simulink model "gm_combinedTxRx_AXIMM"  (R2017b)
settings: Solver=FixedStepDiscrete  StartTime=0.0  StopTime=10.0  RelTol=1e-3
InitFcn:
  | modelSettings
undefined symbols (not defined in the file or in its folder): coeff, filt, j, RadioSampleRate, VibertiTracebackLength, xPreambleSeq
libraries: hdlmdlgenlib x24, simulink x20, dsphdlfiltering x20, hdlsllib x10, dspsigops x5, commseqgen3 x4, commdigbbndpm3 x3, commcrc2 x2, commcnvcod2 x2, commsource2 x1, dspstat3 x1, dspmlti4 x1
(part 3 of 6)

== system gm_combinedTxRx_AXIMM/Combined TX and RX/Receiver HDL/Frame Recover/Barker Locate/Measure Phase Ambiguity ==
  data : Inport  OutDataTypeStr=int16  SampleTime=1e-06
  trigger : Inport  Port=2  SampleTime=1e-06
  validIn : Inport  Port=3  SampleTime=1e-06
  Find Max and Set Output Shift : Subsystem
  HDL Opt Complex FIR4 : Subsystem  mask{Taps=reshape([complex(-0.7071067811865477, -0.7071067811865475) complex(-0.7071067811865477, -0.7071067811865475) complex(-0.7071067811865477, -0.7071067811865475) complex(0.7071067811865476, 0.7071067811865476) complex(0.7071067811865476, 0.7071067811865476) complex(0.7071067811865476, 0.7071067811865476) complex(-0.7071067811865477, -0.7071067811865475) complex(0.7071067811865476, 0.7071067811865476) complex(-0.7071067811865477, -0.7071067811865475) complex(-0.7071067811865477, -0.7071067811865475) complex(0.7071067811865476, 0.7071067811865476) complex(-0.7071067811865477, -0.7071067811865475) complex(-0.7071067811865477, -0.7071067811865475) complex(-0.7071067811865477, -0.7071067811865475) complex(0.7071067811865476, 0.7071067811865476) complex(0.7071067811865476, 0.7071067811865476) complex(0.7071067811865476, 0.7071067811865476) complex(-0.7071067811865477, -0.7071067811865475) complex(0.7071067811865476, 0.7071067811865476) complex(-0.7071067811865477, -0.7071067811865475) complex(-0.7071067811865477, -0.7071067811865475) complex(0.7071067811865476, 0.7071067811865476) complex(-0.7071067811865477, -0.7071067811865475) complex(-0.7071067811865477, -0.7071067811865475) complex(-0.7071067811865477, -0.7071067811865475) complex(0.7071067811865476, 0.7071067811865476) complex(0.7071067811865476, 0.7071067811865476) complex(0.7071067811865476, 0.7071067811865476)].', [1  28])}
  HDL Opt Complex FIR5 : Subsystem  mask{Taps=reshape([complex(-0.7071067811865475, 0.7071067811865477) complex(-0.7071067811865475, 0.7071067811865477) complex(-0.7071067811865475, 0.7071067811865477) complex(0.7071067811865476, -0.7071067811865476) complex(0.7071067811865476, -0.7071067811865476) complex(0.7071067811865476, -0.7071067811865476) complex(-0.7071067811865475, 0.7071067811865477) complex(0.7071067811865476, -0.7071067811865476) complex(-0.7071067811865475, 0.7071067811865477) complex(-0.7071067811865475, 0.7071067811865477) complex(0.7071067811865476, -0.7071067811865476) complex(-0.7071067811865475, 0.7071067811865477) complex(-0.7071067811865475, 0.7071067811865477) complex(-0.7071067811865475, 0.7071067811865477) complex(0.7071067811865476, -0.7071067811865476) complex(0.7071067811865476, -0.7071067811865476) complex(0.7071067811865476, -0.7071067811865476) complex(-0.7071067811865475, 0.7071067811865477) complex(0.7071067811865476, -0.7071067811865476) complex(-0.7071067811865475, 0.7071067811865477) complex(-0.7071067811865475, 0.7071067811865477) complex(0.7071067811865476, -0.7071067811865476) complex(-0.7071067811865475, 0.7071067811865477) complex(-0.7071067811865475, 0.7071067811865477) complex(-0.7071067811865475, 0.7071067811865477) complex(0.7071067811865476, -0.7071067811865476) complex(0.7071067811865476, -0.7071067811865476) complex(0.7071067811865476, -0.7071067811865476)].', [1  28])}
  HDL Opt Complex FIR6 : Subsystem  mask{Taps=reshape([complex(0.7071067811865476, 0.7071067811865476) complex(0.7071067811865476, 0.7071067811865476) complex(0.7071067811865476, 0.7071067811865476) complex(-0.7071067811865475, -0.7071067811865477) complex(-0.7071067811865475, -0.7071067811865477) complex(-0.7071067811865475, -0.7071067811865477) complex(0.7071067811865476, 0.7071067811865476) complex(-0.7071067811865475, -0.7071067811865477) complex(0.7071067811865476, 0.7071067811865476) complex(0.7071067811865476, 0.7071067811865476) complex(-0.7071067811865475, -0.7071067811865477) complex(0.7071067811865476, 0.7071067811865476) complex(0.7071067811865476, 0.7071067811865476) complex(0.7071067811865476, 0.7071067811865476) complex(-0.7071067811865475, -0.7071067811865477) complex(-0.7071067811865475, -0.7071067811865477) complex(-0.7071067811865475, -0.7071067811865477) complex(0.7071067811865476, 0.7071067811865476) complex(-0.7071067811865475, -0.7071067811865477) complex(0.7071067811865476, 0.7071067811865476) complex(0.7071067811865476, 0.7071067811865476) complex(-0.7071067811865475, -0.7071067811865477) complex(0.7071067811865476, 0.7071067811865476) complex(0.7071067811865476, 0.7071067811865476) complex(0.7071067811865476, 0.7071067811865476) complex(-0.7071067811865475, -0.7071067811865477) complex(-0.7071067811865475, -0.7071067811865477) complex(-0.7071067811865475, -0.7071067811865477)].', [1  28])}
  HDL Opt Complex FIR7 : Subsystem  mask{Taps=reshape([complex(0.7071067811865476, -0.7071067811865476) complex(0.7071067811865476, -0.7071067811865476) complex(0.7071067811865476, -0.7071067811865476) complex(-0.7071067811865477, 0.7071067811865475) complex(-0.7071067811865477, 0.7071067811865475) complex(-0.7071067811865477, 0.7071067811865475) complex(0.7071067811865476, -0.7071067811865476) complex(-0.7071067811865477, 0.7071067811865475) complex(0.7071067811865476, -0.7071067811865476) complex(0.7071067811865476, -0.7071067811865476) complex(-0.7071067811865477, 0.7071067811865475) complex(0.7071067811865476, -0.7071067811865476) complex(0.7071067811865476, -0.7071067811865476) complex(0.7071067811865476, -0.7071067811865476) complex(-0.7071067811865477, 0.7071067811865475) complex(-0.7071067811865477, 0.7071067811865475) complex(-0.7071067811865477, 0.7071067811865475) complex(0.7071067811865476, -0.7071067811865476) complex(-0.7071067811865477, 0.7071067811865475) complex(0.7071067811865476, -0.7071067811865476) complex(0.7071067811865476, -0.7071067811865476) complex(-0.7071067811865477, 0.7071067811865475) complex(0.7071067811865476, -0.7071067811865476) complex(0.7071067811865476, -0.7071067811865476) complex(0.7071067811865476, -0.7071067811865476) complex(-0.7071067811865477, 0.7071067811865475) complex(-0.7071067811865477, 0.7071067811865475) complex(-0.7071067811865477, 0.7071067811865475)].', [1  28])}
  Logical Operator : Logic  Inputs=5  AllPortsSameDT=off  OutDataTypeStr=boolean  SampleTime=1e-06
  delayMatch{,1..3} (4 alike) : Delay  DelayLength=hex2num('4010000000000000')  InitialCondition=0  InputProcessing=Inherited  SampleTime=1e-06
  PA : Outport  InitialOutput=0
  wires:
  Find Max and Set Output Shift/1(Out1) -> PA/1
  HDL Opt Complex FIR4/1(Out1) -> Find Max and Set Output Shift/1(In1)
  delayMatch/1 -> Logical Operator/1
  HDL Opt Complex FIR5/1(Out1) -> Find Max and Set Output Shift/2(In2)
  delayMatch1/1 -> Logical Operator/2
  HDL Opt Complex FIR6/1(Out1) -> Find Max and Set Output Shift/3(In4)
  delayMatch2/1 -> Logical Operator/3
  HDL Opt Complex FIR7/1(Out1) -> Find Max and Set Output Shift/4(In5)
  delayMatch3/1 -> Logical Operator/4
  Logical Operator/1 -> Find Max and Set Output Shift/5(Enable)
  data/1 -> HDL Opt Complex FIR4/1(In1), HDL Opt Complex FIR5/1(In1), HDL Opt Complex FIR7/1(In1), HDL Opt Complex FIR6/1(In1)
  trigger/1 -> Logical Operator/5
  validIn/1 -> HDL Opt Complex FIR4/2(validIn), HDL Opt Complex FIR5/2(validIn), HDL Opt Complex FIR7/2(validIn), HDL Opt Complex FIR6/2(validIn)
  HDL Opt Complex FIR4/2(validOut) -> delayMatch/1
  HDL Opt Complex FIR5/2(validOut) -> delayMatch1/1
  HDL Opt Complex FIR6/2(validOut) -> delayMatch2/1
  HDL Opt Complex FIR7/2(validOut) -> delayMatch3/1

== system gm_combinedTxRx_AXIMM/Combined TX and RX/Receiver HDL/Frame Recover/Equalization and Demodulation/2 Bit Descrambler ==
  note: This is a special Descrambler which can process 2 bits at a time
  u1 : Inport  PortDimensions=2  SampleTime=1e-06
  reset : Inport  Port=2  SampleTime=1e-06
  Enable_out4 : Inport  Port=3  OutDataTypeStr=boolean  SampleTime=1e-06
  MATLAB Function : Subsystem
      settings: MinAlgLoopOccurrences=on
  Selector1 : Selector  SampleTime=1e-06  IndexOptions=Index vector (dialog)  Indices=[hex2num('3ff0000000000000') hex2num('4008000000000000') hex2num('4014000000000000') hex2num('401c000000000000')]  OutputSizes=hex2num('3ff0000000000000')
  Selector2 : Selector  SampleTime=1e-06  IndexOptions=Index vector (dialog)  Indices=[hex2num('3ff0000000000000') hex2num('4008000000000000') hex2num('4014000000000000') hex2num('401c000000000000')]  OutputSizes=hex2num('3ff0000000000000')
  delayMatch : Delay  DelayLength=hex2num('4000000000000000')  InitialCondition=0  InputProcessing=Inherited
  input_xor1 : Logic  Operator=XOR  AllPortsSameDT=off  OutDataTypeStr=boolean  SampleTime=1e-06
  input_xor2 : Logic  Operator=XOR  AllPortsSameDT=off  OutDataTypeStr=boolean  SampleTime=1e-06
  mux : Mux  Inputs=2
  state_xor1 : Logic  Operator=XOR  Inputs=1  AllPortsSameDT=off  OutDataTypeStr=boolean  SampleTime=1e-06
  state_xor2 : Logic  Operator=XOR  Inputs=1  AllPortsSameDT=off  OutDataTypeStr=boolean  SampleTime=1e-06
  t : Demux  Outputs=2
  u1_0_wire : hdlmdlgenlib/Buffer
      settings: SourceProductName=HDL Coder  SourceProductBaseCode=HD
  u1_1_wire : hdlmdlgenlib/Buffer
      settings: SourceProductName=HDL Coder  SourceProductBaseCode=HD
  y1 : Outport  InitialOutput=0
  wires:
  u1_0_wire/1 -> input_xor1/2
  u1_1_wire/1 -> input_xor2/2
  MATLAB Function/1(out0) -> Selector1/1
  MATLAB Function/2(out1) -> Selector2/1
  mux/1 -> y1/1
  Selector1/1 -> state_xor1/1
  Selector2/1 -> state_xor2/1
  input_xor1/1 -> mux/1
  input_xor2/1 -> mux/2
  state_xor1/1 -> input_xor1/1
  state_xor2/1 -> input_xor2/1
  delayMatch/1 -> MATLAB Function/Enable
  t/1 -> u1_0_wire/1
  t/2 -> u1_1_wire/1
  u1/1 -> t/1, MATLAB Function/1(in0)
  reset/1 -> MATLAB Function/2(in1)
  Enable_out4/1 -> delayMatch/1

== system gm_combinedTxRx_AXIMM/Combined TX and RX/Receiver HDL/Frame Recover/Equalization and Demodulation/Align with Start ==
  in0 : Inport  OutDataTypeStr=boolean  SampleTime=1e-06
  Enable_out4 : EnablePort  OutDataTypeStr=boolean
  Align with Start : Delay  DelayLength=hex2num('3ff0000000000000')  InitialCondition=0  InputProcessing=Inherited
  out0 : Outport  OutDataTypeStr=boolean  InitialOutput=0
  wires:
  Align with Start/1 -> out0/1
  in0/1 -> Align with Start/1

== system gm_combinedTxRx_AXIMM/Combined TX and RX/Receiver HDL/Frame Recover/Equalization and Demodulation/DFE ==
  note: Generate training sequence when barker is found
  note: refTap=0 to disableEQ
  Trigger : Inport  PortDimensions=1  SampleTime=1e-06
  data : Inport  Port=2  PortDimensions=1  SampleTime=1e-06
      settings: SignalType=complex
  EQmu : Inport  Port=3  SampleTime=1e-06
  Enable_out4 : Inport  Port=4  OutDataTypeStr=boolean  SampleTime=1e-06
  DFE : Subsystem  mask{numFTaps=hex2num('4014000000000000'), numBTaps=hex2num('4008000000000000'), mu=hex2num('3f847ae147ae147b'), refTap=hex2num('4000000000000000')}
      mask prompts: numFTaps "Num Forward Taps"; numBTaps "Num Backward Taps"; mu "Step Size"; refTap "Reference Tap"
  Delay data so DFE can reset : Subsystem
      settings: MinAlgLoopOccurrences=on
  Delay ref so DFE can reset : Subsystem
      settings: MinAlgLoopOccurrences=on
  PN Sequence Generator : Subsystem
      settings: MinAlgLoopOccurrences=on
  Packeted To Unpacked : Subsystem
  QPSK Modulator Baseband : Subsystem
      settings: MinAlgLoopOccurrences=on
  Terminator1 : Terminator
  delayMatch : Delay  DelayLength=hex2num('4000000000000000')  InitialCondition=0  InputProcessing=Inherited
  dataEQed : Outport  InitialOutput=0
  start : Outport  Port=2  InitialOutput=0
  wires:
  DFE/1(eqOut) -> dataEQed/1
  DFE/2(err) -> Terminator1/1
  DFE/3(start) -> start/1
  Delay data so DFE can reset/1(out0) -> DFE/2(dataIn)
  Delay ref so DFE can reset/1(out0) -> DFE/3(training)
  PN Sequence Generator/1(out0) -> Packeted To Unpacked/1(In1)
  Packeted To Unpacked/1(Out1) -> QPSK Modulator Baseband/1(in0)
  QPSK Modulator Baseband/1(out0) -> Delay ref so DFE can reset/1(in0)
  delayMatch/1 -> Delay data so DFE can reset/Enable
  Trigger/1 -> PN Sequence Generator/1(in0), DFE/1(reset)
  data/1 -> Delay data so DFE can reset/1(in0)
  EQmu/1 -> DFE/4(EQmu)
  Enable_out4/1 -> delayMatch/1, QPSK Modulator Baseband/Enable, PN Sequence Generator/Enable, Delay ref so DFE can reset/Enable, DFE/5(Enable_out4)

== system gm_combinedTxRx_AXIMM/Combined TX and RX/Receiver HDL/Frame Recover/Equalization and Demodulation/Header Controller ==
  in0 : Inport  OutDataTypeStr=boolean  SampleTime=1e-06
  in1 : Inport  Port=2  OutDataTypeStr=boolean  PortDimensions=[2]  SampleTime=1e-06
  Enable_out4 : EnablePort  OutDataTypeStr=boolean
  Header Controller : Subsystem
  out0 : Outport  OutDataTypeStr=boolean  InitialOutput=0
  out1 : Outport  Port=2  OutDataTypeStr=uint16  InitialOutput=0
  out2 : Outport  Port=3  OutDataTypeStr=boolean  InitialOutput=0
  out3 : Outport  Port=4  OutDataTypeStr=boolean  InitialOutput=0
  out4 : Outport  Port=5  OutDataTypeStr=uint8  InitialOutput=0
  out5 : Outport  Port=6  OutDataTypeStr=uint32  InitialOutput=0
  out6 : Outport  Port=7  OutDataTypeStr=uint32  InitialOutput=0
  wires:
  Header Controller/1(enableDownstream) -> out0/1
  Header Controller/2(packetLenBitsOut) -> out1/1
  Header Controller/3(resetViterbi) -> out2/1
  Header Controller/4(crcStart) -> out3/1
  Header Controller/5(status) -> out4/1
  Header Controller/6(s1) -> out5/1
  Header Controller/7(s2) -> out6/1
  in0/1 -> Header Controller/1(headerStart)
  in1/1 -> Header Controller/2(data)

== system gm_combinedTxRx_AXIMM/Combined TX and RX/Receiver HDL/Frame Recover/Equalization and Demodulation/QPSK Demodulator Baseband ==
  in0 : Inport  OutDataTypeStr=fixdt(1, 16, 14)  SampleTime=1e-06
      settings: SignalType=complex
  Enable_out4 : EnablePort  OutDataTypeStr=boolean
  QPSK Demodulator Baseband : commdigbbndpm3/QPSK Demodulator Baseband  OutType=Bit  DecType=Hard decision  VarSource=Dialog  Variance=1  Dec=Binary  Ph=pi/4  outDtype1=boolean  outDtype2=Inherit via internal rule  derotateFactorWordLen=16  derotateFactorDataTypeStr=Inherit: Same word length as input  derotateFactorLastDataTypeStr=Inherit: Same word length as input
  out0 : Outport  OutDataTypeStr=boolean  PortDimensions=[2]  InitialOutput=0
  wires:
  QPSK Demodulator Baseband/1 -> out0/1
  in0/1 -> QPSK Demodulator Baseband/1

== system gm_combinedTxRx_AXIMM/Combined TX and RX/Receiver HDL/Frame Recover/Equalization and Demodulation/Skip EQ Training Symbols After Barker ==
  in0 : Inport  OutDataTypeStr=boolean  SampleTime=1e-06
  Enable_out4 : EnablePort  OutDataTypeStr=boolean
  Skip EQ Training Symbols After Barker : Delay  DelayLength=hex2num('406f400000000000')  InitialCondition=0  InputProcessing=Inherited
  out0 : Outport  OutDataTypeStr=boolean  InitialOutput=0
  wires:
  Skip EQ Training Symbols After Barker/1 -> out0/1
  in0/1 -> Skip EQ Training Symbols After Barker/1

== system gm_combinedTxRx_AXIMM/Combined TX and RX/Receiver HDL/Frame Recover/Frequency Recovery/Delay ==
  in0 : Inport  OutDataTypeStr=fixdt(1, 16, 13)  SampleTime=1e-06
      settings: SignalType=complex
  Enable_out4 : EnablePort  OutDataTypeStr=boolean
  Delay : Delay  DelayLength=hex2num('3ff0000000000000')  InitialCondition=0  InputProcessing=Inherited
  out0 : Outport  OutDataTypeStr=fixdt(1, 16, 13)  InitialOutput=0
      settings: SignalType=complex
  wires:
  Delay/1 -> out0/1
  in0/1 -> Delay/1

== system gm_combinedTxRx_AXIMM/Combined TX and RX/Receiver HDL/Frame Recover/Frequency Recovery/Lock Detector ==
  ped : Inport  SampleTime=1e-06
  Enable_out4 : Inport  Port=2  OutDataTypeStr=boolean  SampleTime=1e-06
  Compare To Constant : simulink/Logic and Bit Operations/Compare To Constant  relop=<=  const=fi(0,0,23,10,'hex','000c00')  OutDataTypeStr=boolean
  MATLAB Function : Subsystem
  Pipeline Delay : Subsystem
      settings: MinAlgLoopOccurrences=on
  Sum of Elements : Sum  Inputs=+  AccumDataTypeStr=fixdt(0, 23, 10)  OutDataTypeStr=fixdt(0, 23, 10)  SampleTime=1e-06
  Tapped Delay : Subsystem
      settings: MinAlgLoopOccurrences=on
  lock : Outport  InitialOutput=0
  wires:
  Compare To Constant/1 -> lock/1
  MATLAB Function/1(y) -> Tapped Delay/1(in0)
  Pipeline Delay/1(out0) -> MATLAB Function/1(u)
  Sum of Elements/1 -> Compare To Constant/1
  Tapped Delay/1(out0) -> Sum of Elements/1
  ped/1 -> Pipeline Delay/1(in0)
  Enable_out4/1 -> Tapped Delay/Enable, Pipeline Delay/Enable

== system gm_combinedTxRx_AXIMM/Combined TX and RX/Receiver HDL/Frame Recover/Frequency Recovery/Loop Filter Configurable ==
  note: This inflation is necessary
  e : Inport  SampleTime=1e-06
  LoopBW : Inport  Port=2  SampleTime=1e-06
  Enable_out4 : Inport  Port=3  OutDataTypeStr=boolean  SampleTime=1e-06
  Add1 : Sum  AccumDataTypeStr=fixdt(1, 17, 10)  OutDataTypeStr=fixdt(1, 16, 10)  RndMeth=Nearest  SampleTime=1e-06
  Add2 : Sum  AccumDataTypeStr=fixdt(1, 17, 10)  OutDataTypeStr=fixdt(1, 16, 10)  SampleTime=1e-06
  Data Type Conversion : DataTypeConversion  OutDataTypeStr=fixdt(1, 25, 20)  SampleTime=1e-06
  Delay : Subsystem
      settings: MinAlgLoopOccurrences=on
  Delay3 : Subsystem
      settings: MinAlgLoopOccurrences=on
  Delay4 : Subsystem
      settings: MinAlgLoopOccurrences=on
  Direct Lookup Table (n-D) : LookupNDDirect  NumberOfTableDimensions=1  Table="reshape([0.038055419921875;0.074676513671875;0.109954833984375;0.143951416015625;0.1767578125;0.208404541015625;0.23895263671875;0.268463134765625;0.296966552734375;0.324554443359375;0.351226806640625;0.3770751953125;0.402069091796875;0.426300048828125;0.44976806640625;0.472564697265625;0.49462890625;0.51605224609375;0.536865234375;0.55706787109375;0.576690673828125;0.59576416015625;0.614288330078125;0.63232421875;0.64984130859375;0.666900634765625;0.683502197265625;0.699676513671875;0.715423583984375;0.730743408203125;0.745697021484375;0.76025390625;0.774444580078125;0.788299560546875;0.801788330078125;0.814971923828125;0.82781982421875;0.840362548828125;0.85260009765625;0.86456298828125;0.876251220703125;0.887664794921875;0.8988037109375;0.909698486328125;0.92034912109375;0.930755615234375;0.94091796875;0.950897216796875;0.96063232421875;0.97015380859375;0.979461669921875;0.98858642578125;0.99749755859375;1.006256103515625;1.014801025390625;1.023162841796875;1.0313720703125;1.0394287109375;1.047271728515625;1.05499267578125;1.06256103515625;1.0699462890625;1.07720947265625;1.084320068359375;1.09130859375;1.09814453125;1.1048583984375;1.111419677734375;1.117889404296875;1.12420654296875;1.130401611328125;1.136505126953125;1.142486572265625;1.148345947265625;1.154083251953125;1.159759521484375;1.165283203125;1.170745849609375;1.17608642578125;1.18133544921875;1.18646240234375;1.1915283203125;1.196502685546875;1.201385498046875;1.2061767578125;1.21087646484375;1.21551513671875;1.220062255859375;1.224517822265625;1.228912353515625;1.23321533203125;1.237457275390625;1.241607666015625;1.2457275390625;1.249725341796875;1.253692626953125;1.257568359375;1.26141357421875;1.265167236328125;1.26885986328125;1.272491455078125;1.27606201171875;1.279571533203125;1.28302001953125;1.286407470703125;1.289764404296875;1.29302978515625;1.2962646484375;1.2994384765625;1.302581787109375;1.3056640625;1.308685302734375;1.3116455078125;1.3145751953125;1.317474365234375;1.3203125;1.323089599609375;1.325836181640625;1.328521728515625;1.3311767578125;1.33380126953125;1.33636474609375;1.338897705078125;1.341400146484375;1.343841552734375;1.34625244140625;1.3486328125;1.350982666015625], [128    1])"  DiagnosticForOutOfRangeInput=Error  SampleTime=1e-06  TableDataTypeStr=fixdt('ufix16_En15')
  Direct Lookup Table (n-D)1 : LookupNDDirect  NumberOfTableDimensions=1  Table="reshape([1.1444091796875e-05;4.482269287109375e-05;0.00010013580322265625;0.00017452239990234375;0.00026798248291015625;0.00037860870361328125;0.00050640106201171875;0.0006504058837890625;0.00080966949462890625;0.00098323822021484375;0.001171112060546875;0.0013713836669921875;0.00158405303955078125;0.00180816650390625;0.002044677734375;0.0022907257080078125;0.0025482177734375;0.00281524658203125;0.00309085845947265625;0.003376007080078125;0.00366973876953125;0.00397205352783203125;0.00428104400634765625;0.0045986175537109375;0.0049228668212890625;0.0052547454833984375;0.00559234619140625;0.00593662261962890625;0.00628662109375;0.0066432952880859375;0.00700473785400390625;0.0073719024658203125;0.00774478912353515625;0.008121490478515625;0.00850391387939453125;0.0088901519775390625;0.009281158447265625;0.00967693328857421875;0.0100765228271484375;0.01047992706298828125;0.01088619232177734375;0.0112972259521484375;0.01171207427978515625;0.0121288299560546875;0.01255035400390625;0.012973785400390625;0.013401031494140625;0.01383113861083984375;0.01426410675048828125;0.01469898223876953125;0.01513671875;0.0155773162841796875;0.01602077484130859375;0.0164661407470703125;0.01691341400146484375;0.0173625946044921875;0.01781463623046875;0.018268585205078125;0.0187244415283203125;0.0191822052001953125;0.01964092254638671875;0.02010250091552734375;0.020565032958984375;0.02102947235107421875;0.021495819091796875;0.0219631195068359375;0.0224323272705078125;0.02290248870849609375;0.02337360382080078125;0.02384662628173828125;0.0243206024169921875;0.02479648590087890625;0.02527332305908203125;0.0257511138916015625;0.0262298583984375;0.02670955657958984375;0.02719020843505859375;0.02767181396484375;0.0281543731689453125;0.02863788604736328125;0.02912235260009765625;0.0296077728271484375;0.030094146728515625;0.0305805206298828125;0.03106784820556640625;0.03155612945556640625;0.0320453643798828125;0.03253459930419921875;0.03302478790283203125;0.03351593017578125;0.03400707244873046875;0.03449916839599609375;0.03499126434326171875;0.03548431396484375;0.03597736358642578125;0.03647136688232421875;0.03696537017822265625;0.03745937347412109375;0.0379543304443359375;0.0384502410888671875;0.03894519805908203125;0.0394420623779296875;0.0399379730224609375;0.04043483734130859375;0.04093170166015625;0.04142856597900390625;0.0419254302978515625;0.042423248291015625;0.0429210662841796875;0.04341888427734375;0.04391765594482421875;0.04441547393798828125;0.04491424560546875;0.04541301727294921875;0.0459117889404296875;0.04641056060791015625;0.046909332275390625;0.04740810394287109375;0.04790782928466796875;0.0484066009521484375;0.0489063262939453125;0.04940509796142578125;0.04990482330322265625;0.05040454864501953125;0.0509033203125;0.051403045654296875;0.05190181732177734375;0.05240154266357421875], [128    1])"  DiagnosticForOutOfRangeInput=Error  SampleTime=1e-06  TableDataTypeStr=fixdt('ufix16_En20')
  Product : Product  Inputs=**  OutDataTypeStr=fixdt(1, 16, 10)  SampleTime=1e-06
  Product1 : Product  Inputs=**  OutDataTypeStr=fixdt(1, 16, 10)  SampleTime=1e-06
  Sum2 : Sum  AccumDataTypeStr=fixdt(1, 17, 10)  OutDataTypeStr=fixdt(1, 16, 10)  SampleTime=1e-06
  v : Outport  InitialOutput=0
  wires:
  e/1 -> Product1/1, Product/1
  LoopBW/1 -> Direct Lookup Table (n-D)1/1, Direct Lookup Table (n-D)/1
  Add1/1 -> Sum2/2
  Add2/1 -> Data Type Conversion/1, Delay4/1(in0)
  Data Type Conversion/1 -> v/1
  Delay/1(out0) -> Add1/1
  Delay3/1(out0) -> Add2/1
  Delay4/1(out0) -> Add2/2
  Direct Lookup Table (n-D)/1 -> Product/2
  Direct Lookup Table (n-D)1/1 -> Product1/2
  Product/1 -> Sum2/1
  Product1/1 -> Add1/2, Delay/1(in0)
  Sum2/1 -> Delay3/1(in0)
  Enable_out4/1 -> Delay4/Enable, Delay3/Enable, Delay/Enable

== system gm_combinedTxRx_AXIMM/Combined TX and RX/Receiver HDL/Frame Recover/Frequency Recovery/PED ==
  In : Inport  SampleTime=1e-06
  RxTxFixedPointLibrary_c16_PED : MATLAB Function  TreatAsAtomicUnit=on
  e : Outport  InitialOutput=0
  wires:
  In/1 -> RxTxFixedPointLibrary_c16_PED/1(In)
  RxTxFixedPointLibrary_c16_PED/1(e) -> e/1

== system gm_combinedTxRx_AXIMM/Combined TX and RX/Receiver HDL/Frame Recover/Frequency Recovery/Phase Shift FP ==
  In1 : Inport  SampleTime=1e-06
  Phi : Inport  Port=2  SampleTime=1e-06
  Cosine HDL Optimized : hdlsllib/Lookup Tables/Cosine HDL Optimized  OutputFormula=exp(j*2*pi*u)  NumDataPoints=256  TableDataTypeStr=fixdt(0,31,20)  SimulateLUTROMDelay=off
      settings: SourceProductName=HDL Coder  SourceProductBaseCode=HD
  Gain : Gain  Gain=fi(0,1,25,20,'hex','1fd741a')  ParamDataTypeStr=fixdt(1, 25, 20)  OutDataTypeStr=fixdt(1, 16, 12)  SampleTime=1e-06  SaturateOnIntegerOverflow=on
  Product{,1..3} (4 alike) : Product  Inputs=**  OutDataTypeStr=fixdt(1, 16, 13)  SampleTime=1e-06  SaturateOnIntegerOverflow=on
  Product_AC_minus_BD : Sum  Inputs=+-  OutDataTypeStr=fixdt(1, 16, 13)  SampleTime=1e-06  SaturateOnIntegerOverflow=on
  Product_AD_plus_BC : Sum  OutDataTypeStr=fixdt(1, 16, 13)  SampleTime=1e-06  SaturateOnIntegerOverflow=on
  Product_C2ReIm_1 : ComplexToRealImag  SampleTime=1e-06
  Product_C2ReIm_2 : ComplexToRealImag  SampleTime=1e-06
  Product_ReIm2Complex : RealImagToComplex  SampleTime=1e-06
  Out1 : Outport  InitialOutput=0
  wires:
  In1/1 -> Product_C2ReIm_1/1
  Phi/1 -> Gain/1
  Cosine HDL Optimized/1 -> Product_C2ReIm_2/1
  Gain/1 -> Cosine HDL Optimized/1
  Product_ReIm2Complex/1 -> Out1/1
  Product_C2ReIm_1/1 -> Product1/1, Product/1
  Product_C2ReIm_1/2 -> Product3/1, Product2/1
  Product_C2ReIm_2/1 -> Product3/2, Product/2
  Product_C2ReIm_2/2 -> Product2/2, Product1/2
  Product/1 -> Product_AC_minus_BD/1
  Product1/1 -> Product_AD_plus_BC/1
  Product2/1 -> Product_AC_minus_BD/2
  Product3/1 -> Product_AD_plus_BC/2
  Product_AC_minus_BD/1 -> Product_ReIm2Complex/1
  Product_AD_plus_BC/1 -> Product_ReIm2Complex/2

== system gm_combinedTxRx_AXIMM/Combined TX and RX/Receiver HDL/Frame Recover/Gardner Timing Recovery/Delay ==
  in0 : Inport  OutDataTypeStr=fixdt(0, 15, 14)  SampleTime=1e-06
  Enable_out2 : EnablePort  OutDataTypeStr=boolean
  Delay : Delay  DelayLength=hex2num('3ff0000000000000')  InitialCondition=0  InputProcessing=Inherited
  out0 : Outport  OutDataTypeStr=fixdt(0, 15, 14)  InitialOutput=0
  wires:
  Delay/1 -> out0/1
  in0/1 -> Delay/1

== system gm_combinedTxRx_AXIMM/Combined TX and RX/Receiver HDL/Frame Recover/Gardner Timing Recovery/Delay1 ==
  in0 : Inport  OutDataTypeStr=boolean  SampleTime=1e-06
  Enable_out2 : EnablePort  OutDataTypeStr=boolean
  Delay1 : Delay  DelayLength=hex2num('3ff0000000000000')  InitialCondition=0  InputProcessing=Inherited
  out0 : Outport  OutDataTypeStr=boolean  InitialOutput=0
  wires:
  Delay1/1 -> out0/1
  in0/1 -> Delay1/1

== system gm_combinedTxRx_AXIMM/Combined TX and RX/Receiver HDL/Frame Recover/Gardner Timing Recovery/Delay2 ==
  in0 : Inport  OutDataTypeStr=fixdt(1, 16, 13)  SampleTime=1e-06
      settings: SignalType=complex
  Enable_out2 : EnablePort  OutDataTypeStr=boolean
  Delay2 : Delay  DelayLength=hex2num('4018000000000000')  InitialCondition=0  InputProcessing=Inherited
  out0 : Outport  OutDataTypeStr=fixdt(1, 16, 13)  InitialOutput=0
      settings: SignalType=complex
  wires:
  Delay2/1 -> out0/1
  in0/1 -> Delay2/1

== system gm_combinedTxRx_AXIMM/Combined TX and RX/Receiver HDL/Frame Recover/Gardner Timing Recovery/Gardner TED Blocks ==
  note: This is for QPSK and 4 SamplesPerSymbol ONLY
  data : Inport  SampleTime=1e-06
  strobe : Inport  Port=2  SampleTime=1e-06
  Enable_out2 : Inport  Port=3  OutDataTypeStr=boolean  SampleTime=1e-06
  Add : Sum  AccumDataTypeStr=fixdt(1, 33, 20)  OutDataTypeStr=fixdt(1, 16, 15)  SampleTime=1e-06
  Check Only Strobe Condition : simulink/Logic and Bit Operations/Compare To Constant  relop===  const=fi(0,1,8,0,'hex','01')  OutDataTypeStr=boolean
  Complex to Real-Imag : ComplexToRealImag  SampleTime=1e-06
  Constant : Constant  Value=fi(0,1,16,15,'hex','0000')  OutDataTypeStr=fixdt(1, 16, 15)  SampleTime=-1
  Display : Display
  Imag Error : Subsystem
  Logical Operator : Logic  AllPortsSameDT=off  OutDataTypeStr=boolean  SampleTime=1e-06
  Map [0,1,2,3,4] to [0,1,2,2,2] : LookupNDDirect  NumberOfTableDimensions=1  Table="reshape([hex2num('0000000000000000') hex2num('3ff0000000000000') hex2num('4000000000000000') hex2num('4000000000000000') hex2num('4000000000000000')].', [1  5])"  DiagnosticForOutOfRangeInput=Error  SampleTime=1e-06  TableDataTypeStr=uint8
  Real Error : Subsystem
  Strobe Buffer1_tap1 : Subsystem
      settings: MinAlgLoopOccurrences=on
  Strobe Buffer1_tap2 : Subsystem
      settings: MinAlgLoopOccurrences=on
  Strobe Buffer1_tap3 : Subsystem
      settings: MinAlgLoopOccurrences=on
  Sum of Elements1 : Sum  Inputs=+  AccumDataTypeStr=fixdt(0, 10, 0)  OutDataTypeStr=int8  SampleTime=1e-06
  Switch : Switch  Criteria=u2 ~= 0  Threshold=hex2num('0000000000000000')  OutDataTypeStr=fixdt(1, 16, 15)  SampleTime=1e-06  SaturateOnIntegerOverflow=on
  t : Mux
  e : Outport  InitialOutput=0
  wires:
  data/1 -> Complex to Real-Imag/1
  strobe/1 -> Logical Operator/2, Strobe Buffer1_tap1/1(in0), t/4
  Add/1 -> Switch/1
  Check Only Strobe Condition/1 -> Logical Operator/1
  Complex to Real-Imag/1 -> Real Error/1(data)
  Complex to Real-Imag/2 -> Imag Error/1(data)
  Constant/1 -> Switch/3
  Imag Error/1(Out1) -> Add/2
  Logical Operator/1 -> Switch/2
  Map [0,1,2,3,4] to [0,1,2,2,2]/1 -> Imag Error/2(strobe sum), Real Error/2(strobe sum)
  Real Error/1(Out1) -> Add/1
  t/1 -> Sum of Elements1/1
  Sum of Elements1/1 -> Map [0,1,2,3,4] to [0,1,2,2,2]/1, Check Only Strobe Condition/1, Display/1
  Switch/1 -> e/1
  Strobe Buffer1_tap1/1(out0) -> Strobe Buffer1_tap2/1(in0), t/3
  Strobe Buffer1_tap2/1(out0) -> Strobe Buffer1_tap3/1(in0), t/2
  Strobe Buffer1_tap3/1(out0) -> t/1
  Enable_out2/1 -> Strobe Buffer1_tap3/Enable, Strobe Buffer1_tap2/Enable, Strobe Buffer1_tap1/Enable, Real Error/3(Enable_out2), Imag Error/3(Enable_out2)

== system gm_combinedTxRx_AXIMM/Combined TX and RX/Receiver HDL/Frame Recover/Gardner Timing Recovery/InterpControl_Blocks1 ==
  note: Mu is always positive
  note: e<<1/SPS
  e : Inport  SampleTime=1e-06
  Enable_out2 : Inport  Port=2  OutDataTypeStr=boolean  SampleTime=1e-06
  1/SPS1 : Constant  Value=fi(0,0,2,2,'hex','1')  OutDataTypeStr=fixdt(0, 2, 2)  SampleTime=-1
  Add1 : Sum  AccumDataTypeStr=fixdt(1, 25, 24)  OutDataTypeStr=fixdt(0, 16, 16)  SampleTime=1e-06
  Calculate New mu : Subsystem
  Display{,1..3} (4 alike) : Display
  Mod 1 : Subsystem
  NCOCounter State : Subsystem
      settings: MinAlgLoopOccurrences=on
  Subtract1 : Sum  Inputs=-+  AccumDataTypeStr=fixdt(1, 17, 16)  OutDataTypeStr=fixdt(0, 16, 16)  SampleTime=1e-06
  Update mu on strobe : Switch  Criteria=u2 > Threshold  Threshold=hex2num('0000000000000000')  OutDataTypeStr=fixdt(0, 15, 14)  SampleTime=1e-06
  saved mu : Subsystem
      settings: MinAlgLoopOccurrences=on
  strobe == W>NCOCounter : RelationalOperator  Operator=>  OutDataTypeStr=boolean  SampleTime=1e-06  RndMeth=Nearest
  strobe : Outport  InitialOutput=0
  mu : Outport  Port=2  InitialOutput=0
  wires:
  e/1 -> Add1/1
  1/SPS1/1 -> Add1/2
  Add1/1 -> strobe == W>NCOCounter/1, Subtract1/1, Display2/1, Calculate New mu/1(W)
  Calculate New mu/1(mu) -> Update mu on strobe/1, Display/1
  Mod 1/1(Out1) -> NCOCounter State/1(in0)
  NCOCounter State/1(out0) -> strobe == W>NCOCounter/2, Subtract1/2, Display1/1, Calculate New mu/2(NCOCounter)
  Subtract1/1 -> Mod 1/1(In1)
  Update mu on strobe/1 -> saved mu/1(in0), Display3/1, mu/1
  saved mu/1(out0) -> Update mu on strobe/3
  strobe == W>NCOCounter/1 -> Update mu on strobe/2, strobe/1
  Enable_out2/1 -> saved mu/Enable, NCOCounter State/Enable

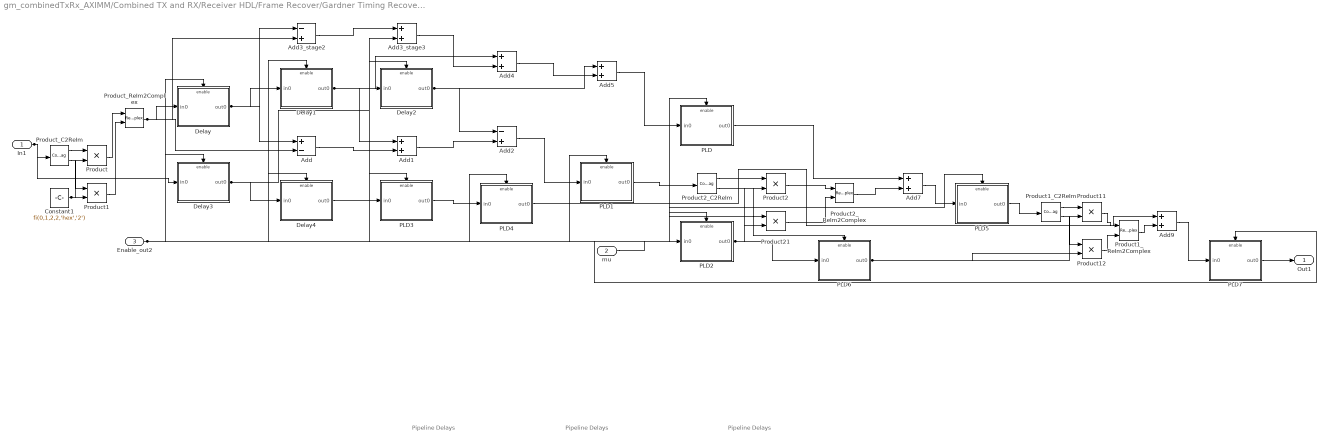
== system gm_combinedTxRx_AXIMM/Combined TX and RX/Receiver HDL/Frame Recover/Gardner Timing Recovery/Interpolator ==
  note: Pipeline Delays
  note: Pipeline Delays
  note: Pipeline Delays
  In1 : Inport  SampleTime=1e-06
  mu : Inport  Port=2  SampleTime=1e-06
  Enable_out2 : Inport  Port=3  OutDataTypeStr=boolean  SampleTime=1e-06
  Add : Sum  Inputs=+-  AccumDataTypeStr=fixdt(1, 17, 14)  OutDataTypeStr=fixdt(1, 16, 14)  SampleTime=1e-06
  Add1 : Sum  AccumDataTypeStr=fixdt(1, 17, 14)  OutDataTypeStr=fixdt(1, 17, 14)  SampleTime=1e-06
  Add2 : Sum  Inputs=-+  AccumDataTypeStr=fixdt(1, 18, 14)  OutDataTypeStr=fixdt(1, 18, 14)  SampleTime=1e-06
  Add3_stage2 : Sum  Inputs=-+  AccumDataTypeStr=fixdt(1, 18, 14)  OutDataTypeStr=fixdt(1, 18, 14)  SampleTime=1e-06
  Add3_stage3 : Sum  AccumDataTypeStr=fixdt(1, 18, 14)  OutDataTypeStr=fixdt(1, 18, 14)  SampleTime=1e-06
  Add4 : Sum  AccumDataTypeStr=fixdt(1, 19, 14)  OutDataTypeStr=fixdt(1, 19, 14)  SampleTime=1e-06
  Add5 : Sum  AccumDataTypeStr=fixdt(1, 20, 14)  OutDataTypeStr=fixdt(1, 20, 14)  SampleTime=1e-06
  Add7 : Sum  AccumDataTypeStr=fixdt(1, 21, 14)  OutDataTypeStr=fixdt(1, 21, 14)  SampleTime=1e-06
  Add9 : Sum  AccumDataTypeStr=fixdt(1, 37, 28)  OutDataTypeStr=fixdt(1, 16, 10)  SampleTime=1e-06
  Constant1 : Constant  Value=fi(0,1,2,2,'hex','2')  OutDataTypeStr=fixdt(1, 2, 2)  SampleTime=-1
  Delay : Subsystem
      settings: MinAlgLoopOccurrences=on
  Delay1 : Subsystem
      settings: MinAlgLoopOccurrences=on
  Delay2 : Subsystem
      settings: MinAlgLoopOccurrences=on
  Delay3 : Subsystem
      settings: MinAlgLoopOccurrences=on
  Delay4 : Subsystem
      settings: MinAlgLoopOccurrences=on
  PLD : Subsystem
      settings: MinAlgLoopOccurrences=on
  PLD1 : Subsystem
      settings: MinAlgLoopOccurrences=on
  PLD2 : Subsystem
      settings: MinAlgLoopOccurrences=on
  PLD3 : Subsystem
      settings: MinAlgLoopOccurrences=on
  PLD4 : Subsystem
      settings: MinAlgLoopOccurrences=on
  PLD5 : Subsystem
      settings: MinAlgLoopOccurrences=on
  PLD6 : Subsystem
      settings: MinAlgLoopOccurrences=on
  PLD7 : Subsystem
      settings: MinAlgLoopOccurrences=on
  Product : Product  Inputs=**  OutDataTypeStr=fixdt(1, 16, 14)  SampleTime=1e-06
  Product1 : Product  Inputs=**  OutDataTypeStr=fixdt(1, 16, 14)  SampleTime=1e-06
  Product11 : Product  Inputs=**  OutDataTypeStr=fixdt(1, 36, 28)  SampleTime=1e-06
  Product12 : Product  Inputs=**  OutDataTypeStr=fixdt(1, 36, 28)  SampleTime=1e-06
  Product1_C2ReIm : ComplexToRealImag  SampleTime=1e-06
  Product1_ReIm2Complex : RealImagToComplex  SampleTime=1e-06
  Product2 : Product  Inputs=**  OutDataTypeStr=fixdt(1, 16, 10)  SampleTime=1e-06
  Product21 : Product  Inputs=**  OutDataTypeStr=fixdt(1, 16, 10)  SampleTime=1e-06
  Product2_C2ReIm : ComplexToRealImag  SampleTime=1e-06
  Product2_ReIm2Complex : RealImagToComplex  SampleTime=1e-06
  Product_C2ReIm : ComplexToRealImag  SampleTime=1e-06
  Product_ReIm2Complex : RealImagToComplex  SampleTime=1e-06
  Out1 : Outport  InitialOutput=0
  wires:
  In1/1 -> Product_C2ReIm/1, Delay3/1(in0)
  mu/1 -> PLD2/1(in0)
  Add/1 -> Add1/2
  Add1/1 -> Add2/2
  Add2/1 -> PLD1/1(in0)
  Add3_stage3/1 -> Add4/2
  Add4/1 -> Add5/2
  Add5/1 -> PLD/1(in0)
  Add7/1 -> PLD5/1(in0)
  Add9/1 -> PLD7/1(in0)
  Constant1/1 -> Product1/2, Product/2
  Delay/1(out0) -> Add3_stage2/1, Add/1, Delay1/1(in0)
  Delay1/1(out0) -> Add4/1, Add1/1, Delay2/1(in0)
  Delay2/1(out0) -> Add5/1, Add2/1
  Delay3/1(out0) -> Add3_stage3/2, Delay4/1(in0)
  Delay4/1(out0) -> PLD3/1(in0)
  PLD/1(out0) -> Add7/1
  PLD1/1(out0) -> Product2_C2ReIm/1
  PLD2/1(out0) -> Product21/2, Product2/2, PLD6/1(in0)
  PLD3/1(out0) -> PLD4/1(in0)
  PLD4/1(out0) -> Add9/1
  PLD5/1(out0) -> Product1_C2ReIm/1
  PLD6/1(out0) -> Product12/2, Product11/2
  PLD7/1(out0) -> Out1/1
  Product_ReIm2Complex/1 -> Add3_stage2/2, Add/2, Delay/1(in0)
  Product1_ReIm2Complex/1 -> Add9/2
  Product2_ReIm2Complex/1 -> Add7/2
  Enable_out2/1 -> PLD7/Enable, PLD6/Enable, PLD5/Enable, PLD4/Enable, PLD3/Enable, PLD2/Enable, PLD1/Enable, PLD/Enable, Delay4/Enable, Delay3/Enable, Delay2/Enable, Delay1/Enable, Delay/Enable
  Add3_stage2/1 -> Add3_stage3/1
  Product_C2ReIm/1 -> Product/1
  Product_C2ReIm/2 -> Product1/1
  Product/1 -> Product_ReIm2Complex/1
  Product1/1 -> Product_ReIm2Complex/2
  Product1_C2ReIm/1 -> Product11/1
  Product1_C2ReIm/2 -> Product12/1
  Product11/1 -> Product1_ReIm2Complex/1
  Product12/1 -> Product1_ReIm2Complex/2
  Product2_C2ReIm/1 -> Product2/1
  Product2_C2ReIm/2 -> Product21/1
  Product2/1 -> Product2_ReIm2Complex/1
  Product21/1 -> Product2_ReIm2Complex/2

== system gm_combinedTxRx_AXIMM/Combined TX and RX/Receiver HDL/Frame Recover/Gardner Timing Recovery/LoopFilter1 ==
  e : Inport  SampleTime=1e-06
  Enable_out2 : Inport  Port=2  OutDataTypeStr=boolean  SampleTime=1e-06
  Delay1 : Subsystem
      settings: MinAlgLoopOccurrences=on
  Delay2 : Subsystem
      settings: MinAlgLoopOccurrences=on
  Proportional Gain : Gain  Gain=fi(0,1,16,23,'hex','9500')  ParamDataTypeStr=fixdt(1, 16, 23)  OutDataTypeStr=fixdt(1, 16, 24)  SampleTime=1e-06
  v : Outport  InitialOutput=0
  wires:
  e/1 -> Delay2/1(in0)
  Delay1/1(out0) -> v/1
  Delay2/1(out0) -> Proportional Gain/1
  Proportional Gain/1 -> Delay1/1(in0)
  Enable_out2/1 -> Delay2/Enable, Delay1/Enable

== system gm_combinedTxRx_AXIMM/Combined TX and RX/Receiver HDL/Frame Recover/Gardner Timing Recovery/TED Lock Detector ==
  ted : Inport  SampleTime=1e-06
  Enable_out2 : Inport  Port=2  OutDataTypeStr=boolean  SampleTime=1e-06
  Compare To Constant : simulink/Logic and Bit Operations/Compare To Constant  relop=<=  const=fi(0,0,23,15,'hex','008000')  OutDataTypeStr=boolean
  MATLAB Function : Subsystem
  Pipeline Delay : Subsystem
      settings: MinAlgLoopOccurrences=on
  Sum of Elements : Sum  Inputs=+  AccumDataTypeStr=fixdt(0, 23, 15)  OutDataTypeStr=fixdt(0, 23, 15)  SampleTime=1e-06
  Tapped Delay : Subsystem
      settings: MinAlgLoopOccurrences=on
  lock : Outport  InitialOutput=0
  wires:
  Compare To Constant/1 -> lock/1
  MATLAB Function/1(y) -> Tapped Delay/1(in0)
  Pipeline Delay/1(out0) -> MATLAB Function/1(u)
  Sum of Elements/1 -> Compare To Constant/1
  Tapped Delay/1(out0) -> Sum of Elements/1
  ted/1 -> Pipeline Delay/1(in0)
  Enable_out2/1 -> Tapped Delay/Enable, Pipeline Delay/Enable

== system gm_combinedTxRx_AXIMM/Combined TX and RX/Receiver HDL/Viterbi Decode/Buffer/MATLAB Function ==
  valid : Inport  SampleTime=1e-06
  start : Inport  Port=2  SampleTime=1e-06
  crcEnd : Inport  Port=3  SampleTime=1e-06
  RxTxFixedPointLibrary_c26_MATLAB_Function : MATLAB Function  TreatAsAtomicUnit=on
  enable : Outport
  wires:
  RxTxFixedPointLibrary_c26_MATLAB_Function/1(enable) -> enable/1
  valid/1 -> RxTxFixedPointLibrary_c26_MATLAB_Function/1(valid)
  start/1 -> RxTxFixedPointLibrary_c26_MATLAB_Function/2(start)
  crcEnd/1 -> RxTxFixedPointLibrary_c26_MATLAB_Function/3(crcEnd)

== system gm_combinedTxRx_AXIMM/Combined TX and RX/Receiver HDL/Viterbi Decode/Buffer/MATLAB Function1 ==
  packetLen : Inport  SampleTime=1e-06
  valid : Inport  Port=2  SampleTime=1e-06
  crcStart : Inport  Port=3  SampleTime=1e-06
  RxTxFixedPointLibrary_c2_MATLAB_Function1 : MATLAB Function  TreatAsAtomicUnit=on
  enablePop : Outport
  validOut : Outport  Port=2
  viterbiReset : Outport  Port=3
  crcOut : Outport  Port=4
  wires:
  RxTxFixedPointLibrary_c2_MATLAB_Function1/1(enablePop) -> enablePop/1
  RxTxFixedPointLibrary_c2_MATLAB_Function1/2(validOut) -> validOut/1
  RxTxFixedPointLibrary_c2_MATLAB_Function1/3(viterbiReset) -> viterbiReset/1
  RxTxFixedPointLibrary_c2_MATLAB_Function1/4(crcOut) -> crcOut/1
  packetLen/1 -> RxTxFixedPointLibrary_c2_MATLAB_Function1/1(packetLen)
  valid/1 -> RxTxFixedPointLibrary_c2_MATLAB_Function1/2(valid)
  crcStart/1 -> RxTxFixedPointLibrary_c2_MATLAB_Function1/3(crcStart)

== system gm_combinedTxRx_AXIMM/Combined TX and RX/Transmitter HDL/Packet Generation/Payload/HDL Scrambler 2 bits ==
  bitsIn : Inport  PortDimensions=[2, 1]  SampleTime=4e-06
  reset : Inport  Port=2  SampleTime=4e-06
  Buffer Manage : Subsystem
  Delay : Delay  DelayLength=1  InitialCondition=false
  Delay1 : Delay  DelayLength=1  InitialCondition=false
  Demux : Demux  Outputs=2
  Display1 : Display
  Display3 : Display
  Mux : Mux  Inputs=2
  Mux1 : Mux  Inputs=2
  Selector : Selector  IndexOptions=Index vector (dialog)  Indices=find(poly(2:end))  OutputSizes=1
  Selector1 : Selector  IndexOptions=Index vector (dialog)  Indices=1+find(poly(2:end))  OutputSizes=1
  state_xor1 : Logic  Operator=XOR  IconShape=distinctive  AllPortsSameDT=off  OutDataTypeStr=boolean
  state_xor2 : Logic  Operator=XOR  Inputs=1  IconShape=distinctive  AllPortsSameDT=off  OutDataTypeStr=boolean
  state_xor3 : Logic  Operator=XOR  Inputs=1  IconShape=distinctive  AllPortsSameDT=off  OutDataTypeStr=boolean
  state_xor4 : Logic  Operator=XOR  IconShape=distinctive  AllPortsSameDT=off  OutDataTypeStr=boolean
  bitsOut : Outport
  wires:
  bitsIn/1 -> Demux/1, Display1/1
  reset/1 -> Buffer Manage/3(reset)
  Buffer Manage/1(outBuffer) -> Selector/1, Mux1/1
  Delay/1 -> Buffer Manage/1(bit1)
  Delay1/1 -> Buffer Manage/2(bit2)
  Demux/1 -> state_xor1/2
  Demux/2 -> state_xor4/2
  Mux/1 -> bitsOut/1
  Mux1/1 -> Selector1/1
  Selector/1 -> state_xor2/1
  Selector1/1 -> state_xor3/1
  state_xor1/1 -> Mux1/2, Mux/1, Delay/1
  state_xor2/1 -> state_xor1/1, Display3/1
  state_xor3/1 -> state_xor4/1
  state_xor4/1 -> Mux/2, Delay1/1

== system gm_combinedTxRx_AXIMM/Combined TX and RX/Transmitter HDL/Packet Generation/Payload/MATLAB Function ==
  enable : Inport  SampleTime=4e-06
  RxTxFixedPointLibrary_c4_MATLAB_Function : MATLAB Function  TreatAsAtomicUnit=on
  reset : Outport
  mode : Outport  Port=2
  wires:
  enable/1 -> RxTxFixedPointLibrary_c4_MATLAB_Function/1(enable)
  RxTxFixedPointLibrary_c4_MATLAB_Function/1(reset) -> reset/1
  RxTxFixedPointLibrary_c4_MATLAB_Function/2(mode) -> mode/1

== system gm_combinedTxRx_AXIMM/Combined TX and RX/Transmitter HDL/Packet Generation/Payload/Subsystem ==
  In1 : Inport  SampleTime=4e-06
  In2 : Inport  Port=2  SampleTime=4e-06
  Logical Operator : Logic  Operator=OR  Inputs=3  AllPortsSameDT=off  OutDataTypeStr=boolean
  MATLAB Function3 : Subsystem
  Out1 : Outport
  wires:
  In1/1 -> Logical Operator/1, MATLAB Function3/1(start)
  In2/1 -> Logical Operator/3, MATLAB Function3/2(done)
  Logical Operator/1 -> Out1/1
  MATLAB Function3/1(enable) -> Logical Operator/2

== system gm_combinedTxRx_AXIMM/Combined TX and RX/Transmitter HDL/Packet Generation/Preamble/Unpack1 ==
  In1 : Inport  SampleTime=4e-06
  Data Type Conversion : DataTypeConversion  OutDataTypeStr=boolean
  Extract Bits : simulink/Logic and Bit Operations/Extract Bits  bitsToExtract=Range of bits  numBits=8  bitIdxRange=[1]  outScalingMode=Treat bit field as an integer
      settings: SourceProductName=Simulink
  Extract Bits1 : simulink/Logic and Bit Operations/Extract Bits  bitsToExtract=Range of bits  numBits=8  bitIdxRange=[0]  outScalingMode=Treat bit field as an integer
      settings: SourceProductName=Simulink
  Vector Concatenate : Concatenate
  Out1 : Outport
  wires:
  Data Type Conversion/1 -> Out1/1
  Extract Bits/1 -> Vector Concatenate/1
  Extract Bits1/1 -> Vector Concatenate/2
  Vector Concatenate/1 -> Data Type Conversion/1
  In1/1 -> Extract Bits1/1, Extract Bits/1

== system gm_combinedTxRx_AXIMM/Combined TX and RX/Transmitter HDL/Packet Generation/Random Data/Unpack ==
  In1 : Inport  SampleTime=4e-06
  Data Type Conversion : DataTypeConversion  OutDataTypeStr=boolean
  Extract Bits : simulink/Logic and Bit Operations/Extract Bits  bitsToExtract=Range of bits  numBits=8  bitIdxRange=[0]  outScalingMode=Treat bit field as an integer
      settings: SourceProductName=Simulink
  Extract Bits1 : simulink/Logic and Bit Operations/Extract Bits  bitsToExtract=Range of bits  numBits=8  bitIdxRange=[1]  outScalingMode=Treat bit field as an integer
      settings: SourceProductName=Simulink
  Vector Concatenate : Concatenate
  Out1 : Outport
  wires:
  In1/1 -> Extract Bits1/1, Extract Bits/1
  Data Type Conversion/1 -> Out1/1
  Extract Bits/1 -> Vector Concatenate/1
  Extract Bits1/1 -> Vector Concatenate/2
  Vector Concatenate/1 -> Data Type Conversion/1

== system gm_combinedTxRx_AXIMM/Combined TX and RX/Receiver HDL/Frame Recover/Barker Locate/Measure Phase Ambiguity/Find Max and Set Output Shift ==
  In1 : Inport  SampleTime=1e-06
  In2 : Inport  Port=2  SampleTime=1e-06
  In4 : Inport  Port=3  SampleTime=1e-06
  In5 : Inport  Port=4  SampleTime=1e-06
  Enable : Inport  Port=5  OutDataTypeStr=boolean  SampleTime=1e-06
  Complex to Real-Imag{,1..3} (4 alike) : ComplexToRealImag  Output=Imag  SampleTime=1e-06
  Direct Lookup Table (n-D) : LookupNDDirect  NumberOfTableDimensions=1  Table="reshape([complex(1, 0) complex(6.123233995736766e-17, -1) complex(-1, -1.2246467991473532e-16) complex(-1.8369701987210297e-16, 1)].', [4  1])"  DiagnosticForOutOfRangeInput=Error  SampleTime=1e-06  TableDataTypeStr=fixdt(1,16,13)
  Direct Lookup Table (n-D)_out1_bypass : hdlmdlgenlib/Buffer
      settings: SourceProductName=HDL Coder  SourceProductBaseCode=HD
  Display : Display
  Display1 : Display
  Maximum : dspstat3/Maximum  operation=maximum  fcn=Index  indexBase=Zero  operateOver=Each column  Dimension=1  InputProcessing=Columns as channels (frame based)  reset=None  roiEnable=off  roiType=Rectangles  roiPortion=Entire ROI  roiOutput=Individual statistics for each ROI  roiFlag=off  roundingMode=Floor  overflowMode=off  accumDataTypeStr=Inherit: Same as product output  accumLastDataTypeStr=Inherit: Same as product output
  Out1_bypass : UnitDelay  SampleTime=1e-06
  PipelineRegister : Delay  DelayLength=hex2num('3ff0000000000000')  InitialCondition=0  InputProcessing=Inherited
  concatenate : Concatenate  NumInputs=4
  concatenate1 : Concatenate  NumInputs=4
  delayMatch : Delay  DelayLength=hex2num('4008000000000000')  InitialCondition=0  InputProcessing=Inherited
  t : MultiPortSwitch  DataPortOrder=Zero-based contiguous  Inputs=2  zeroidx=on  OutDataTypeStr=fixdt(1, 16, 13)  SampleTime=1e-06
  Out1 : Outport  InitialOutput=0
  wires:
  Complex to Real-Imag/1 -> concatenate/1
  Complex to Real-Imag1/1 -> concatenate/2
  Complex to Real-Imag2/1 -> concatenate/3
  Complex to Real-Imag3/1 -> concatenate/4
  delayMatch/1 -> t/3
  Maximum/1 -> Direct Lookup Table (n-D)/1
  concatenate/1 -> Display/1, Maximum/1
  concatenate1/1 -> Display1/1
  Direct Lookup Table (n-D)_out1_bypass/1 -> Out1/1
  In1/1 -> concatenate1/1, Complex to Real-Imag/1
  In2/1 -> concatenate1/2, Complex to Real-Imag1/1
  In4/1 -> concatenate1/3, Complex to Real-Imag2/1
  In5/1 -> concatenate1/4, Complex to Real-Imag3/1
  Enable/1 -> t/1
  PipelineRegister/1 -> delayMatch/1
  Out1_bypass/1 -> t/2
  t/1 -> Direct Lookup Table (n-D)_out1_bypass/1, Out1_bypass/1
  Direct Lookup Table (n-D)/1 -> PipelineRegister/1
